simulink model "Q2sim"  (R2022a)
settings: Solver=VariableStepAuto  StartTime=ts  StopTime=tf  FixedStep=tstep  RelTol=1e-3
settings Model: Creator=nsm0014  LastModifiedBy=nsm0014

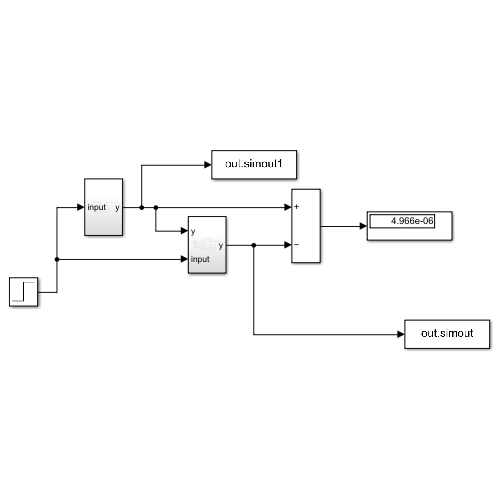
[thumbnail: Simulink's stored preview of the top-level diagram]
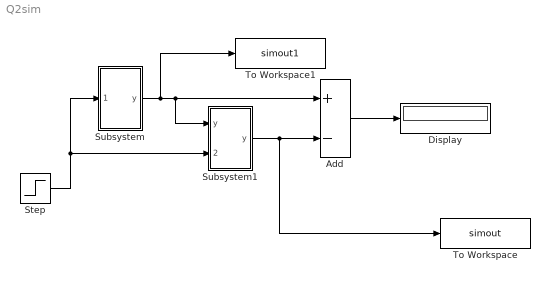
== system Q2sim ==
  Add : Sum  Inputs=+-
  Display : Display
  Step : Step  SampleTime=0
  Subsystem : Subsystem
  Subsystem1 : Subsystem
  To Workspace : ToWorkspace  VariableName=simout  SaveFormat=Structure With Time  SampleTime=-1
  To Workspace1 : ToWorkspace  VariableName=simout1  SaveFormat=Structure With Time  SampleTime=-1
  wires:
  Subsystem/1(y) -> To Workspace1/1, Subsystem1/1("y "), Add/1
  Subsystem1/1(y) -> To Workspace/1, Add/2
  Add/1 -> Display/1
  Step/1 -> Subsystem1/2(input), Subsystem/1(input)

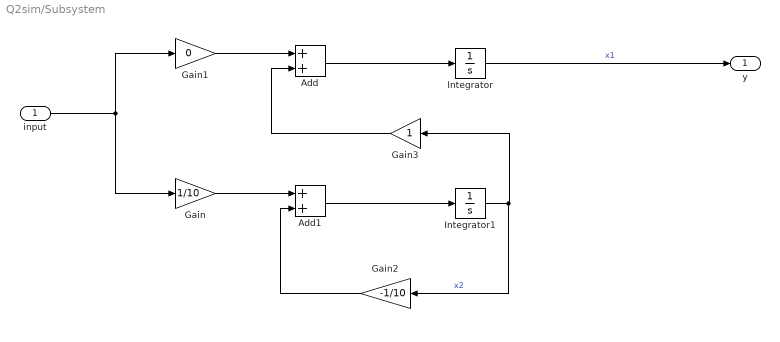
== system Q2sim/Subsystem ==
  input : Inport
  Add : Sum
  Add1 : Sum
  Gain : Gain  Gain=1/10
  Gain1 : Gain  Gain=0
  Gain2 : Gain  Gain=-1/10
  Gain3 : Gain
  Integrator : Integrator
  Integrator1 : Integrator
  y : Outport
  wires:
  Gain1/1 -> Add/1
  Integrator/1 -> y/1  "x1"
  Integrator1/1 -> Gain3/1, Gain2/1  "x2"
  Gain/1 -> Add1/1
  Gain2/1 -> Add1/2
  input/1 -> Gain/1, Gain1/1
  Add1/1 -> Integrator1/1
  Add/1 -> Integrator/1
  Gain3/1 -> Add/2

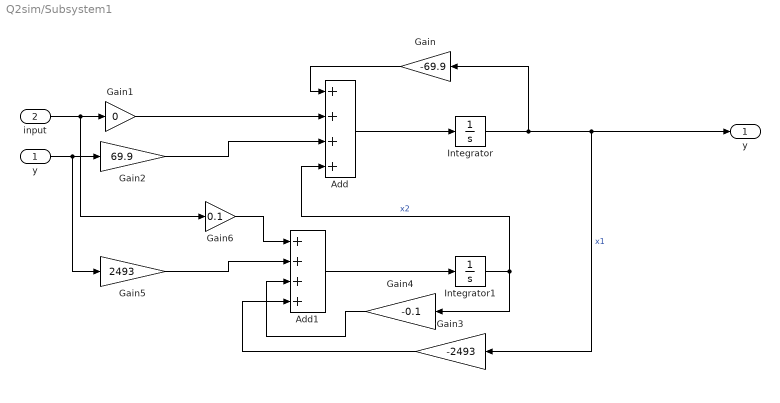
== system Q2sim/Subsystem1 ==
  "y " : Inport
  input : Inport  Port=2
  Add : Sum  Inputs=++++
  Add1 : Sum  Inputs=++++
  Gain : Gain  Gain=-69.9
  Gain1 : Gain  Gain=0
  Gain2 : Gain  Gain=69.9
  Gain3 : Gain  Gain=-2493
  Gain4 : Gain  Gain=-0.1
  Gain5 : Gain  Gain=2493
  Gain6 : Gain  Gain=0.1
  Integrator : Integrator
  Integrator1 : Integrator
  y : Outport
  wires:
  Integrator1/1 -> Add/4, Gain4/1  "x2"
  Integrator/1 -> Gain/1, Gain3/1, y/1  "x1"
  Add/1 -> Integrator/1
  Gain/1 -> Add/1
  input/1 -> Gain6/1, Gain1/1
  Gain1/1 -> Add/2
  Gain2/1 -> Add/3
  "y "/1 -> Gain5/1, Gain2/1
  Gain6/1 -> Add1/1
  Gain5/1 -> Add1/2
  Gain4/1 -> Add1/3
  Gain3/1 -> Add1/4
  Add1/1 -> Integrator1/1
